simulink model "PolePlacement2024_Liftoff_HW"  (R2025b)
settings: Solver=ode1  StartTime=0.0  StopTime=inf  FixedStep=0.002  RelTol=1e-3  EnableMultiTasking=on
PreLoadFcn:
  | if exist('data/liftoff_params.mat','file'), load('data/liftoff_params.mat'); end
PostLoadFcn:
  | qc_set_target_type(getConfigSet(bdroot, 'QUARC Default Target Configuration'));
undefined symbols (not defined in the file): c_catch, HIL, K_lift, Kf, P_lyap
libraries: quarc_library x4
settings Model: SimulationMode=external  ExtModeTrigDuration=5000  Creator=pmartin  LastModifiedBy=U448565
settings SolverCC: AlgebraicLoopSolver=TrustRegion  PositivePriorityOrder=on
settings DataIOCC: LimitDataPoints=on  SaveFormat=Array  SignalLoggingSaveFormat=ModelDataLogs  ReturnWorkspaceOutputs=off
settings OptimizationCC: ExpressionDepthLimit=2147483647.0  InitFltsAndDblsToZero=on
settings DebuggingCC: SaveWithParameterizedLinksMsg=none  UnderspecifiedInitializationDetection=Classic  MergeDetectMultiDrivingBlocksExec=none  SolverPrmCheckMsg=warning  MultiTaskDSMMsg=warning  MultiTaskCondExecSysMsg=none  FcnCallInpInsideContextMsg=warning  UnconnectedInputMsg=warning  UnconnectedOutputMsg=warning  UnconnectedLineMsg=warning  StateNameClashWarn=warning  SFUnexpectedBacktrackingDiag=warning  SFNoUnconditionalDefaultTransitionDiag=warning  SFExecutionAtInitializationDiag=none  ArithmeticOperatorsInVariantConditions=warning
settings ModelReferenceCC: PropagateSignalLabelsOutOfModel=off
settings SFSimCC: SimUseLocalCustomCode=off  CustomCodeUndefinedFunction=UseInterfaceOnly
settings RTWCC: SystemTargetFile=quarc_win64.tlc  TemplateMakefile=quarc_default_tmf  RTWUseLocalCustomCode=off  Toolchain=QUARC win64 | nmake (64-bit Windows)  BuildConfiguration=Faster Runs  GPUComputeCapability=3.5  Description=QUARC Win64 Target Using Toolchain
settings CodeAppCC: StateflowObjectComments=on
settings STFCustomTargetCC: SystemTargetFile=quarc_win64.tlc  UseToolchainInfoCompliant=on
settings GRTTargetCC: ExtMode=on  ExtModeMexFile=quarc_comm  TargetLangStandard=C89/C90 (ANSI)  ParMdlRefBuildCompliant=off  CompOptLevelCompliant=off  CombineOutputUpdateFcns=off  MatFileLogging=off  CPPClassGenCompliant=off  GRTInterface=on
settings ConfigComp: CovMetricSettings=dw  CovSaveCumulativeToWorkspaceVar=on  CovSaveSingleToWorkspaceVar=on  CovExternalEMLEnable=off

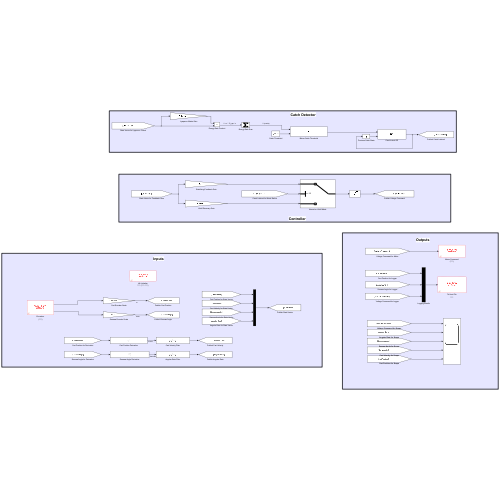
[thumbnail: Simulink's stored preview of the top-level diagram]
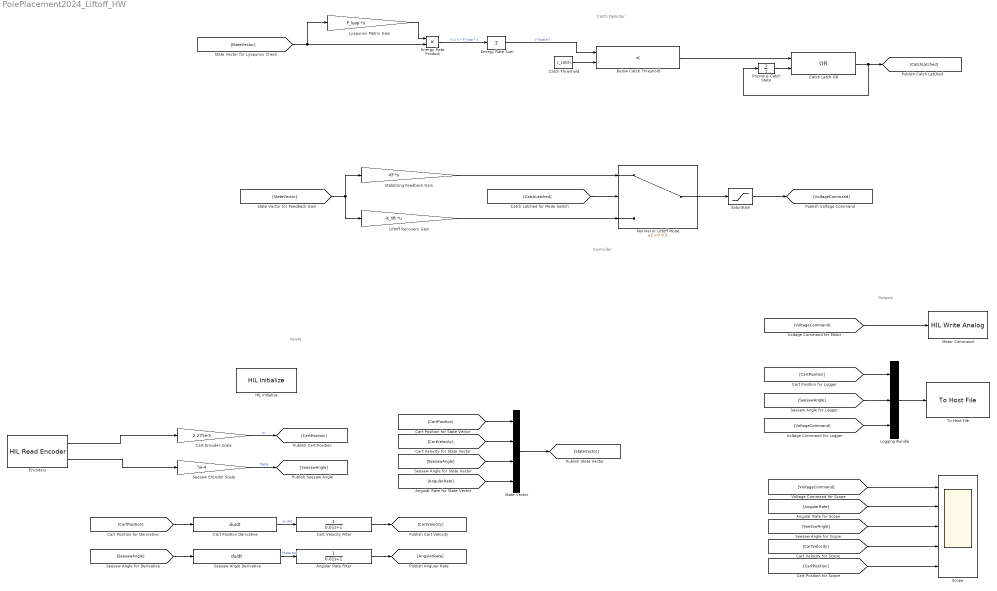
== system PolePlacement2024_Liftoff_HW ==
  note: Catch Detector
  note: Controller
  note: Outputs
  note: Inputs
  Angular Rate Filter : TransferFcn  Denominator=[0.01 1]
  Below Catch Threshold : RelationalOperator  Operator=<  OutDataTypeStr=boolean  RndMeth=Simplest  InputSameDT=off
  Cart Encoder Scale : Gain  Gain=2.275e-5
  Cart Position Derivative : Derivative
  Cart Velocity Filter : TransferFcn  Denominator=[0.01 1]
  Catch Latch OR : Logic  Operator=OR  AllPortsSameDT=off  OutDataTypeStr=boolean
  Catch Threshold : Constant  Value=c_catch
  Encoders : quarc_library/Data Acquisition/Generic/Immediate I//O/HIL Read Encoder  object_name=HIL-1  channels=[0:1]  sample_time=qc_get_step_size  active=on  vector_output=off  data_type_mode=Inherit via back propagation  data_type=double
  Energy Rate Product : Product
  Energy Rate Sum : Sum  Inputs=+
  HIL Initialize : quarc_library/Data Acquisition/Generic/Configuration/HIL Initialize  object_name=HIL-1  board_type=q2_usb  board_number=0  board_options=d0=digital;d1=digital;led=auto;update_rate=normal  exclusive=off  active=off  hardware_clocks=[0:2]  clock_modes=[]  initial_clock_frequencies=[]  set_clock_params_at_start=off  set_clock_params_at_switch_in=off  set_clock_frequencies_at_start=off  set_clock_frequencies_at_switch_in=off  analog_input_channels=[0:1]  analog_input_configurations=[]  analog_input_maximums=10  analog_input_minimums=-10  set_analog_input_params_at_start=on  set_analog_input_params_at_switch_in=off  analog_output_channels=[0:1]  analog_output_maximums=10  analog_output_minimums=-10  initial_analog_outputs=[0]  final_analog_outputs=[0]  watchdog_analog_outputs=0  set_analog_output_params_at_start=on  set_analog_output_params_at_switch_in=off  set_analog_outputs_at_start=on  set_analog_outputs_at_switch_in=off  set_analog_outputs_at_terminate=on  set_analog_outputs_at_switch_out=off  set_analog_outputs_on_watchdog=off  digital_input_channels=[]  digital_output_channels=[0:7]  digital_output_configuration=[]  initial_digital_outputs=[0]  final_digital_outputs=[0]  watchdog_digital_outputs=[0]  set_digital_output_params_at_start=off  set_digital_output_params_at_switch_in=off  set_digital_outputs_at_start=on  set_digital_outputs_at_switch_in=off  set_digital_outputs_at_terminate=on  set_digital_outputs_at_switch_out=off  set_digital_outputs_on_watchdog=off  encoder_channels=[0:1]  quadrature=[4]  encoder_filter_frequency=[]  initial_encoder_counts=[0]  set_encoder_params_at_start=on  set_encoder_params_at_switch_in=off  set_encoder_counts_at_start=on  set_encoder_counts_at_switch_in=off  pwm_channels=[]  pwm_modes=[0]  pwm_frequency=1/0.020  pwm_configuration=[]  pwm_alignment=[]  pwm_polarity=[]  pwm_leading_deadband=[]  pwm_trailing_deadband=[]  initial_pwm_outputs=[0]  final_pwm_outputs=[0]  watchdog_pwm_outputs=[0]  set_pwm_params_at_start=on  set_pwm_params_at_switch_in=off  set_pwm_outputs_at_start=on  set_pwm_outputs_at_switch_in=off  set_pwm_outputs_at_terminate=on  set_pwm_outputs_at_switch_out=off  set_pwm_outputs_on_watchdog=off  other_output_channels=[]  initial_other_outputs=[]  final_other_outputs=[]  watchdog_other_outputs=[]  set_other_outputs_at_start=off  set_other_outputs_at_switch_in=off  set_other_outputs_at_terminate=off  set_other_outputs_at_switch_out=off  set_other_outputs_on_watchdog=off
  Liftoff Recovery Gain : Gain  Gain=-K_lift  Multiplication=Matrix(K*u)
  Logging Bundle : Mux  Inputs=3
  Lyapunov Matrix Gain : Gain  Gain=P_lyap  Multiplication=Matrix(K*u)
  Motor Command : quarc_library/Data Acquisition/Generic/Immediate I//O/HIL Write Analog  object_name=HIL-1  channels=0  sample_time=-1  active=off  vector_input=off
  Normal or Liftoff Mode : Switch  Threshold=0.5  SaturateOnIntegerOverflow=off  InputSameDT=off
  Previous Catch State : UnitDelay  SampleTime=-1  HasFrameUpgradeWarning=on
  Saturation : Saturate  UpperLimit=7  LowerLimit=-7
  Scope : Scope  NumInputPorts=5
      settings: ActiveDisplayYMinimum=-0.89623  ActiveDisplayYMaximum=1.37236
  Seesaw Angle Derivative : Derivative
  Seesaw Encoder Scale : Gain  Gain=5e-4
  Stabilizing Feedback Gain : Gain  Gain=-Kf  Multiplication=Matrix(K*u)
  State Vector : Mux
  To Host File : quarc_library/Sinks/To Host/To Host File  source=Specify via dialog (do not evaluate)  file_name=data_%{date}_%{time}.mat  variable_name=data  decimation=1  sample_time=-1  file_format=MAT-file v.4  options=No header or footer  append=off  final_file_name=data_05-May-2026_17-28-00.mat  encoding=Default  bitrate=0
  wires:
  [AngularRate] -> Scope/2
  [VoltageCommand] -> Logging Bundle/3
  [VoltageCommand] -> Scope/1
  [SeesawAngle] -> Scope/3
  [CartPosition] -> Scope/5
  [SeesawAngle] -> Seesaw Angle Derivative/1
  [SeesawAngle] -> State Vector/3
  [CartVelocity] -> Scope/4
  Catch Latch OR/1 -> Previous Catch State/1, [CatchLatched]
  Liftoff Recovery Gain/1 -> Normal or Liftoff Mode/3
  Encoders/2 -> Seesaw Encoder Scale/1
  Encoders/1 -> Cart Encoder Scale/1
  [VoltageCommand] -> Motor Command/1
  Below Catch Threshold/1 -> Catch Latch OR/1
  [CartPosition] -> Cart Position Derivative/1
  [SeesawAngle] -> Logging Bundle/2
  [CartPosition] -> Logging Bundle/1
  [StateVector] -> Energy Rate Product/2, Lyapunov Matrix Gain/1
  [StateVector] -> Stabilizing Feedback Gain/1, Liftoff Recovery Gain/1
  [CartPosition] -> State Vector/1
  Lyapunov Matrix Gain/1 -> Energy Rate Product/1
  [CartVelocity] -> State Vector/2
  [CatchLatched] -> Normal or Liftoff Mode/2
  [AngularRate] -> State Vector/4
  Seesaw Angle Derivative/1 -> Angular Rate Filter/1  "theta dot"
  Energy Rate Sum/1 -> Below Catch Threshold/1  "V (scalar)"
  Cart Encoder Scale/1 -> [CartPosition]  "xc"
  Energy Rate Product/1 -> Energy Rate Sum/1  "V = x' * P_lyap * x"
  Seesaw Encoder Scale/1 -> [SeesawAngle]  "theta"
  Cart Position Derivative/1 -> Cart Velocity Filter/1  "xc dot"
  Logging Bundle/1 -> To Host File/1
  Stabilizing Feedback Gain/1 -> Normal or Liftoff Mode/1
  State Vector/1 -> [StateVector]
  Angular Rate Filter/1 -> [AngularRate]
  Cart Velocity Filter/1 -> [CartVelocity]
  Catch Threshold/1 -> Below Catch Threshold/2
  Normal or Liftoff Mode/1 -> Saturation/1
  Previous Catch State/1 -> Catch Latch OR/2
  Saturation/1 -> [VoltageCommand]
